simulink model "generic_truck"  (Simulink 8.7)
settings: Solver=ode45  StartTime=0.0  StopTime=inf  RelTol=1e-3
libraries: TruckMaker4SL x1, simulink x1
(part 1 of 2)
settings Model: Creator=fh  LastModifiedBy=IPG  ExtModeAutoUpdateStatusClock=off
settings DataIOCC: SignalLoggingSaveFormat=ModelDataLogs  SignalLoggingName=sigsOut
settings OptimizationCC: BooleanDataType=off  ExpressionDepthLimit=2147483647  InitFltsAndDblsToZero=on
settings DebuggingCC: SaveWithParameterizedLinksMsg=none  SignalResolutionControl=TryResolveAllWithWarning  MultiTaskDSMMsg=warning  MultiTaskCondExecSysMsg=none  FcnCallInpInsideContextMsg=UseLocalSettings  StateNameClashWarn=warning
settings HardwareCC: TargetUnknown=on
settings CodeAppCC: MaxIdLength=63
settings GRTTargetCC: TargetFcnLib=ansi_tfl_tmw.mat  CombineOutputUpdateFcns=off  GRTInterface=on

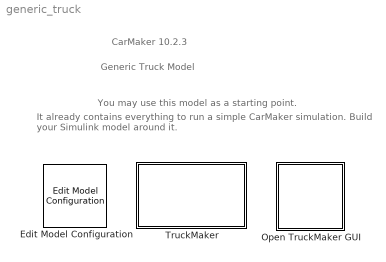
== system generic_truck ==
  note: Generic Truck Model
  note: CarMaker 10.2.3
  note: You may use this model as a starting point.
  note: It already contains everything to run a simple CarMaker simulation.
      | Build your Simulink model around it.
  Edit Model Configuration : TruckMaker4SL/Edit Model Configuration
  Open TruckMaker GUI : Subsystem  LoadFcn=if ~length(which('cmself')), cmenv; end
      settings: OpenFcn=cmblockmagic('gui_fix_display'); TM_Simulink
      mask Display: image(imread('TruckMakerGUI.png'));
  TruckMaker : Subsystem  TreatAsAtomicUnit=on
      mask Display: image(imread('TruckMakerSys.png'));

== system generic_truck/Open TruckMaker GUI ==
  S-Function : S-Function  FunctionName=cm_gui  SFunctionDeploymentMode=off  EnableBusSupport=off

== system generic_truck/TruckMaker ==
  CM_FIRST : Subsystem
  CM_LAST : Subsystem
  DrivMan : Subsystem
  Ground : Ground
  IPG Vehicle : Subsystem  TreatAsAtomicUnit=on
  Terminator : Terminator
  VehicleControl : Subsystem
  wires:
  VehicleControl/2(Vhcl.Model.Source) -> IPG Vehicle/2(Vhcl.Model.Source)
  VehicleControl/7(VhclCtrl.PT) -> IPG Vehicle/7(VhclCtrl.PT)
  VehicleControl/6(VhclCtrl.Brake) -> IPG Vehicle/6(VhclCtrl.Brake)
  VehicleControl/5(Vhcl.Misc) -> IPG Vehicle/5(Vhcl.Misc)
  VehicleControl/4(Vhcl.Wheel.In) -> IPG Vehicle/4(Vhcl.Wheel.In)
  VehicleControl/3(VhclCtrl.Steering) -> IPG Vehicle/3(VhclCtrl.Steering)
  VehicleControl/1(Sync_Out) -> IPG Vehicle/1(Sync_In)
  IPG Vehicle/1(Sync_Out) -> CM_LAST/1(Sync_In)
  Ground/1 -> CM_FIRST/1(Sync_In)
  CM_LAST/1(Sync_Out) -> Terminator/1
  CM_FIRST/1(Sync_Out) -> DrivMan/1(Sync_In)
  CM_FIRST/2(Env.Misc) -> DrivMan/2(Env.Misc)
  DrivMan/1(Sync_Out) -> VehicleControl/1(Sync_In)
  DrivMan/2(DrivMan.Out) -> VehicleControl/2(DrivMan.In)

== system generic_truck/TruckMaker/CM_FIRST ==
  Sync_In : Inport
  BusCreator1 : BusCreator  Inputs=8
  BusCreator2 : BusCreator  Inputs=6
  Demux1 : Demux  Outputs=14
  Environment : S-Function  FunctionName=TM_Sfun  Parameters='Environment'  SFunctionDeploymentMode=off  EnableBusSupport=off
  IoIn : S-Function  FunctionName=TM_Sfun  Parameters='IoIn'  SFunctionDeploymentMode=off  EnableBusSupport=off
  Terminator : Terminator
  Sync_Out : Outport
  Env.Misc : Outport  Port=2
  wires:
  BusCreator2/1 -> Terminator/1  "IF Environment (in)"
  BusCreator1/1 -> Env.Misc/1
  Demux1/14 -> BusCreator2/6  "Env sRoad"
  Demux1/13 -> BusCreator2/5  "Env PoI_GCS Elev"
  Demux1/12 -> BusCreator2/4  "Env PoI_GCS Lat"
  Demux1/11 -> BusCreator2/3  "Env PoI_GCS Long"
  Demux1/10 -> BusCreator2/2  "Env Time"
  Demux1/9 -> BusCreator2/1  "Env yDay"
  Demux1/8 -> BusCreator1/8  "Env WindVel_tot z"
  Demux1/7 -> BusCreator1/7  "Env WindVel_tot y"
  Demux1/6 -> BusCreator1/6  "Env WindVel_tot x"
  Demux1/5 -> BusCreator1/5  "Env SolarRadiation"
  Demux1/4 -> BusCreator1/4  "Env AirHumidity"
  Demux1/3 -> BusCreator1/3  "Env AirPressure"
  Demux1/2 -> BusCreator1/2  "Env AirDensity"
  Demux1/1 -> BusCreator1/1  "Env Temperature"
  Environment/2 -> Demux1/1
  Environment/1 -> Sync_Out/1
  IoIn/1 -> Environment/1
  Sync_In/1 -> IoIn/1

== system generic_truck/TruckMaker/CM_LAST ==
  Sync_In : Inport
  CM_User : S-Function  FunctionName=TM_Sfun  Parameters='CM_User'  SFunctionDeploymentMode=off  EnableBusSupport=off
  IoOut : S-Function  FunctionName=TM_Sfun  Parameters='IoOut'  SFunctionDeploymentMode=off  EnableBusSupport=off
  Sync_Out : Outport
  wires:
  IoOut/1 -> Sync_Out/1
  CM_User/1 -> IoOut/1
  Sync_In/1 -> CM_User/1

== system generic_truck/TruckMaker/DrivMan ==
  note: There's rarely a reason to override DrivMan signals.
      | Use the VehicleControl interface for this purpose.
  Sync_In : Inport
  Env.Misc : Inport  Port=2
  BusCreator : BusCreator  Inputs=17
  Demux : Demux  Outputs=17
  DrivMan : S-Function  FunctionName=TM_Sfun  Parameters='DrivMan'  SFunctionDeploymentMode=off  EnableBusSupport=off
  Sync_Out : Outport
  DrivMan.Out : Outport  Port=2
  wires:
  Demux/17 -> BusCreator/17  "DrivMan Steering Trq"
  Demux/16 -> BusCreator/16  "DrivMan Steering AngAcc"
  Demux/15 -> BusCreator/15  "DrivMan Steering AngVel"
  Demux/14 -> BusCreator/14  "DrivMan Steering Ang"
  Demux/13 -> BusCreator/13  "DrivMan Gas"
  Demux/12 -> BusCreator/12  "DrivMan Clutch"
  Demux/11 -> BusCreator/11  "DrivMan BrakePark"
  Demux/10 -> BusCreator/10  "DrivMan Brake"
  Demux/9 -> BusCreator/9  "DrivMan GearNo"
  Demux/8 -> BusCreator/8  "DrivMan SelectorCtrl"
  Demux/7 -> BusCreator/7  "DrivMan UserSignal4"
  Demux/6 -> BusCreator/6  "DrivMan UserSignal3"
  Demux/5 -> BusCreator/5  "DrivMan UserSignal2"
  Demux/4 -> BusCreator/4  "DrivMan UserSignal1"
  Demux/3 -> BusCreator/3  "DrivMan UserSignal0"
  Demux/2 -> BusCreator/2  "DrivMan Key"
  Demux/1 -> BusCreator/1  "DrivMan SST"
  Env.Misc/1 -> DrivMan/2
  Sync_In/1 -> DrivMan/1
  DrivMan/1 -> Sync_Out/1
  BusCreator/1 -> DrivMan.Out/1
  DrivMan/2 -> Demux/1

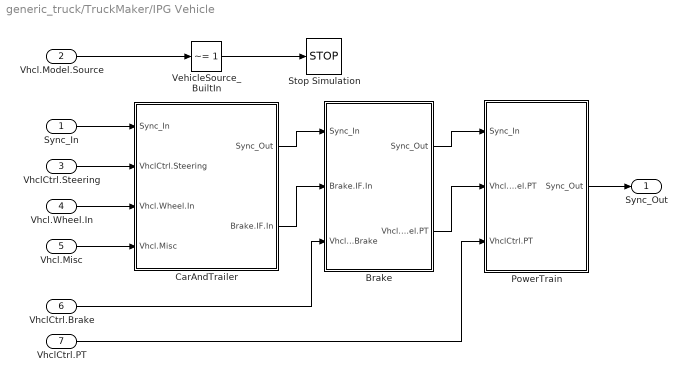
== system generic_truck/TruckMaker/IPG Vehicle ==
  Sync_In : Inport
  Vhcl.Model.Source : Inport  Port=2
  VhclCtrl.Steering : Inport  Port=3
  Vhcl.Wheel.In : Inport  Port=4
  Vhcl.Misc : Inport  Port=5
  VhclCtrl.Brake : Inport  Port=6
  VhclCtrl.PT : Inport  Port=7
  Brake : Subsystem
  CarAndTrailer : Subsystem
  PowerTrain : Subsystem
  Stop Simulation : Stop
  VehicleSource_BuiltIn : simulink/Logic and Bit Operations/Compare To Constant  relop=~=  const=1  OutDataTypeStr=boolean  ZeroCross=off
  Sync_Out : Outport
  wires:
  VhclCtrl.PT/1 -> PowerTrain/3(VhclCtrl.PT)
  Brake/1(Sync_Out) -> PowerTrain/1(Sync_In)
  CarAndTrailer/1(Sync_Out) -> Brake/1(Sync_In)
  CarAndTrailer/2(Brake.IF.In) -> Brake/2(Brake.IF.In)
  VhclCtrl.Brake/1 -> Brake/3(VhclCtrl.Brake)
  PowerTrain/1(Sync_Out) -> Sync_Out/1
  Vhcl.Misc/1 -> CarAndTrailer/4(Vhcl.Misc)
  Vhcl.Wheel.In/1 -> CarAndTrailer/3(Vhcl.Wheel.In)
  VhclCtrl.Steering/1 -> CarAndTrailer/2(VhclCtrl.Steering)
  Sync_In/1 -> CarAndTrailer/1(Sync_In)
  Vhcl.Model.Source/1 -> VehicleSource_BuiltIn/1
  VehicleSource_BuiltIn/1 -> Stop Simulation/1
  Brake/2(Vhcl.Wheel.PT) -> PowerTrain/2(Vhcl.Wheel.PT)

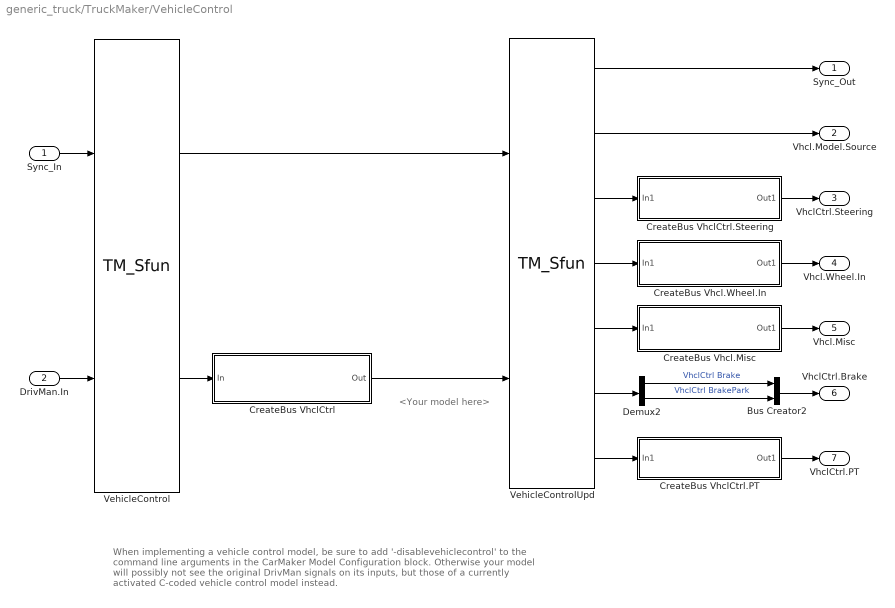
== system generic_truck/TruckMaker/VehicleControl ==
  note: <Your model here>
  note: When implementing a vehicle control model,
      | be sure to add '-disablevehiclecontrol' to the command line arguments
      | in the CarMaker Model Configuration block.
      | Otherwise your model will possibly not see the original DrivMan signals
      | on its inputs, but those of a currently activated C-coded vehicle control model instead.
  Sync_In : Inport
  DrivMan.In : Inport  Port=2
  Bus Creator2 : BusCreator  Inputs=2
  CreateBus Vhcl.Misc : Subsystem
  CreateBus Vhcl.Wheel.In : Subsystem
  CreateBus VhclCtrl : Subsystem
  CreateBus VhclCtrl.PT : Subsystem
  CreateBus VhclCtrl.Steering : Subsystem
  Demux2 : Demux  Outputs=2
  VehicleControl : S-Function  FunctionName=TM_Sfun  Parameters='VehicleControl'  SFunctionDeploymentMode=off  EnableBusSupport=off
  VehicleControlUpd : S-Function  FunctionName=TM_Sfun  Parameters='VehicleControlUpd'  SFunctionDeploymentMode=off  EnableBusSupport=off
  Sync_Out : Outport
  Vhcl.Model.Source : Outport  Port=2
  VhclCtrl.Steering : Outport  Port=3
  Vhcl.Wheel.In : Outport  Port=4
  Vhcl.Misc : Outport  Port=5
  VhclCtrl.Brake : Outport  Port=6
  VhclCtrl.PT : Outport  Port=7
  wires:
  VehicleControlUpd/2 -> Vhcl.Model.Source/1
  VehicleControlUpd/4 -> CreateBus Vhcl.Wheel.In/1(In1)
  VehicleControlUpd/5 -> CreateBus Vhcl.Misc/1(In1)
  VehicleControlUpd/6 -> Demux2/1
  VehicleControlUpd/7 -> CreateBus VhclCtrl.PT/1(In1)
  VehicleControlUpd/3 -> CreateBus VhclCtrl.Steering/1(In1)
  CreateBus Vhcl.Misc/1(Out1) -> Vhcl.Misc/1
  CreateBus Vhcl.Wheel.In/1(Out1) -> Vhcl.Wheel.In/1
  DrivMan.In/1 -> VehicleControl/2
  CreateBus VhclCtrl/1(Out) -> VehicleControlUpd/2
  VehicleControl/1 -> VehicleControlUpd/1
  VehicleControl/2 -> CreateBus VhclCtrl/1(In)
  Sync_In/1 -> VehicleControl/1
  CreateBus VhclCtrl.PT/1(Out1) -> VhclCtrl.PT/1
  Bus Creator2/1 -> VhclCtrl.Brake/1
  CreateBus VhclCtrl.Steering/1(Out1) -> VhclCtrl.Steering/1
  VehicleControlUpd/1 -> Sync_Out/1
  Demux2/2 -> Bus Creator2/2  "VhclCtrl BrakePark"
  Demux2/1 -> Bus Creator2/1  "VhclCtrl Brake"

== system generic_truck/TruckMaker/IPG Vehicle/Brake ==
  note: <Your model here>
  note: When replacing the entire braking system,
      | be sure to disable the IPG brake model by using the brake
      | model 'Model Manager off' in the vehicle GUI.
  Sync_In : Inport
  Brake.IF.In : Inport  Port=2
  VhclCtrl.Brake : Inport  Port=3
  Brake : S-Function  FunctionName=TM_Sfun  Parameters='Brake'  SFunctionDeploymentMode=off  EnableBusSupport=off
  BrakeUpd : S-Function  FunctionName=TM_Sfun  Parameters='BrakeUpd'  SFunctionDeploymentMode=off  EnableBusSupport=off
  BusCreator : BusCreator  Inputs=32
  CreateBus Vhcl.Wheel.PT : Subsystem
  Demux : Demux  Outputs=32
  Sync_Out : Outport
  Vhcl.Wheel.PT : Outport  Port=2
  wires:
  Demux/32 -> BusCreator/32  "Brake IF Trq_DriveSrc_trg d7"
  Demux/31 -> BusCreator/31  "Brake IF Trq_DriveSrc_trg d6"
  Demux/30 -> BusCreator/30  "Brake IF Trq_DriveSrc_trg d5"
  Demux/29 -> BusCreator/29  "Brake IF Trq_DriveSrc_trg d4"
  Demux/28 -> BusCreator/28  "Brake IF Trq_DriveSrc_trg d3"
  Demux/27 -> BusCreator/27  "Brake IF Trq_DriveSrc_trg d2"
  Demux/26 -> BusCreator/26  "Brake IF Trq_DriveSrc_trg d1"
  Demux/25 -> BusCreator/25  "Brake IF Trq_DriveSrc_trg d0"
  Demux/24 -> BusCreator/24  "Brake IF Trq_Reg_trg FR2"
  Demux/23 -> BusCreator/23  "Brake IF Trq_Reg_trg FL2"
  Demux/22 -> BusCreator/22  "Brake IF Trq_Reg_trg RR2"
  Demux/21 -> BusCreator/21  "Brake IF Trq_Reg_trg RL2"
  Demux/20 -> BusCreator/20  "Brake IF Trq_Reg_trg RR"
  Demux/19 -> BusCreator/19  "Brake IF Trq_Reg_trg RL"
  Demux/18 -> BusCreator/18  "Brake IF Trq_Reg_trg FR"
  Demux/17 -> BusCreator/17  "Brake IF Trq_Reg_trg FL"
  Demux/16 -> BusCreator/16  "Brake IF Trq_PB FR2"
  Demux/15 -> BusCreator/15  "Brake IF Trq_PB FL2"
  Demux/14 -> BusCreator/14  "Brake IF Trq_PB RR2"
  Demux/13 -> BusCreator/13  "Brake IF Trq_PB RL2"
  Demux/12 -> BusCreator/12  "Brake IF Trq_PB RR"
  Demux/11 -> BusCreator/11  "Brake IF Trq_PB RL"
  Demux/10 -> BusCreator/10  "Brake IF Trq_PB FR"
  Demux/9 -> BusCreator/9  "Brake IF Trq_PB FL"
  Demux/8 -> BusCreator/8  "Brake IF Trq_WB FR2"
  Demux/7 -> BusCreator/7  "Brake IF Trq_WB FL2"
  Demux/6 -> BusCreator/6  "Brake IF Trq_WB RR2"
  Demux/5 -> BusCreator/5  "Brake IF Trq_WB RL2"
  Demux/4 -> BusCreator/4  "Brake IF Trq_WB RR"
  Demux/3 -> BusCreator/3  "Brake IF Trq_WB RL"
  Demux/2 -> BusCreator/2  "Brake IF Trq_WB FR"
  Demux/1 -> BusCreator/1  "Brake IF Trq_WB FL"
  BusCreator/1 -> BrakeUpd/2
  Brake/2 -> Demux/1
  BrakeUpd/1 -> Sync_Out/1
  Brake/1 -> BrakeUpd/1  "Sync"
  Brake.IF.In/1 -> Brake/2
  VhclCtrl.Brake/1 -> Brake/3
  Sync_In/1 -> Brake/1
  BrakeUpd/2 -> CreateBus Vhcl.Wheel.PT/1(In)
  CreateBus Vhcl.Wheel.PT/1(Out) -> Vhcl.Wheel.PT/1

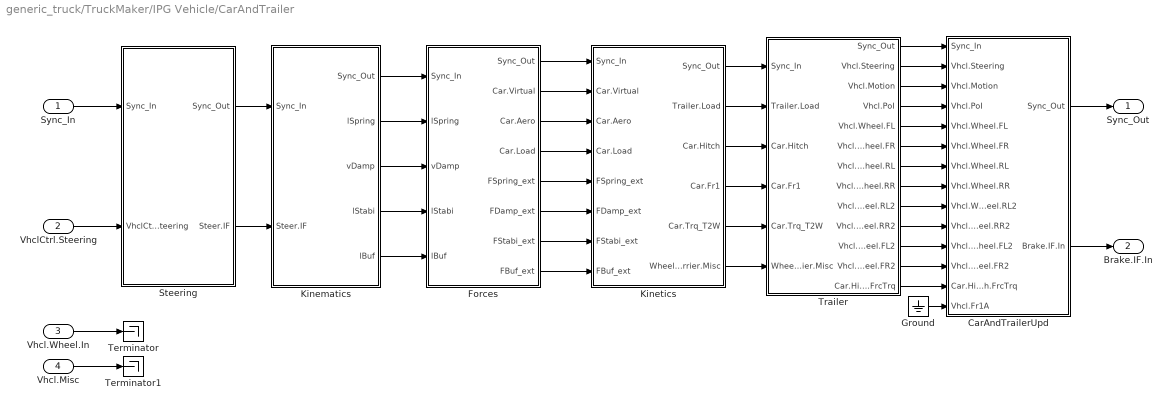
== system generic_truck/TruckMaker/IPG Vehicle/CarAndTrailer ==
  Sync_In : Inport
  VhclCtrl.Steering : Inport  Port=2
  Vhcl.Wheel.In : Inport  Port=3
  Vhcl.Misc : Inport  Port=4
  CarAndTrailerUpd : Subsystem
  Forces : Subsystem
  Ground : Ground
  Kinematics : Subsystem
  Kinetics : Subsystem
  Steering : Subsystem
  Terminator : Terminator
  Terminator1 : Terminator
  Trailer : Subsystem
  Sync_Out : Outport
  Brake.IF.In : Outport  Port=2
  wires:
  Ground/1 -> CarAndTrailerUpd/14(Vhcl.Fr1A)
  Trailer/13(Car.Hitch.FrcTrq) -> CarAndTrailerUpd/13(Car.Hitch.FrcTrq)
  Trailer/12(Vhcl.Wheel.FR2) -> CarAndTrailerUpd/12(Vhcl.Wheel.FR2)
  Trailer/11(Vhcl.Wheel.FL2) -> CarAndTrailerUpd/11(Vhcl.Wheel.FL2)
  Trailer/10(Vhcl.Wheel.RR2) -> CarAndTrailerUpd/10(Vhcl.Wheel.RR2)
  Trailer/9(Vhcl.Wheel.RL2) -> CarAndTrailerUpd/9(Vhcl.Wheel.RL2)
  Trailer/8(Vhcl.Wheel.RR) -> CarAndTrailerUpd/8(Vhcl.Wheel.RR)
  Trailer/7(Vhcl.Wheel.RL) -> CarAndTrailerUpd/7(Vhcl.Wheel.RL)
  Trailer/6(Vhcl.Wheel.FR) -> CarAndTrailerUpd/6(Vhcl.Wheel.FR)
  Trailer/5(Vhcl.Wheel.FL) -> CarAndTrailerUpd/5(Vhcl.Wheel.FL)
  Trailer/4(Vhcl.PoI) -> CarAndTrailerUpd/4(Vhcl.PoI)
  Trailer/3(Vhcl.Motion) -> CarAndTrailerUpd/3(Vhcl.Motion)
  Trailer/2(Vhcl.Steering) -> CarAndTrailerUpd/2(Vhcl.Steering)
  Trailer/1(Sync_Out) -> CarAndTrailerUpd/1(Sync_In)
  CarAndTrailerUpd/2(Brake.IF.In) -> Brake.IF.In/1
  CarAndTrailerUpd/1(Sync_Out) -> Sync_Out/1
  Vhcl.Misc/1 -> Terminator1/1
  Vhcl.Wheel.In/1 -> Terminator/1
  Kinetics/6(WheelCarrier.Misc) -> Trailer/6(WheelCarrier.Misc)
  Kinetics/5(Car.Trq_T2W) -> Trailer/5(Car.Trq_T2W)
  Steering/2(Steer.IF) -> Kinematics/2(Steer.IF)
  Kinetics/4(Car.Fr1) -> Trailer/4(Car.Fr1)
  Kinetics/3(Car.Hitch) -> Trailer/3(Car.Hitch)
  Kinetics/2(Trailer.Load) -> Trailer/2(Trailer.Load)
  VhclCtrl.Steering/1 -> Steering/2(VhclCtrl.Steering)
  Sync_In/1 -> Steering/1(Sync_In)
  Steering/1(Sync_Out) -> Kinematics/1(Sync_In)
  Kinetics/1(Sync_Out) -> Trailer/1(Sync_In)
  Kinematics/5(lBuf) -> Forces/5(lBuf)
  Forces/8(FBuf_ext) -> Kinetics/8(FBuf_ext)
  Forces/4(Car.Load) -> Kinetics/4(Car.Load)
  Forces/7(FStabi_ext) -> Kinetics/7(FStabi_ext)
  Forces/6(FDamp_ext) -> Kinetics/6(FDamp_ext)
  Forces/5(FSpring_ext) -> Kinetics/5(FSpring_ext)
  Forces/2(Car.Virtual) -> Kinetics/2(Car.Virtual)
  Kinematics/2(lSpring) -> Forces/2(lSpring)
  Kinematics/3(vDamp) -> Forces/3(vDamp)
  Forces/3(Car.Aero) -> Kinetics/3(Car.Aero)
  Forces/1(Sync_Out) -> Kinetics/1(Sync_In)
  Kinematics/1(Sync_Out) -> Forces/1(Sync_In)
  Kinematics/4(lStabi) -> Forces/4(lStabi)

== system generic_truck/TruckMaker/IPG Vehicle/PowerTrain ==
  note: When replacing the entire powertrain,
      | be sure to disable the IPG powertrain model by using the powertrain
      | model 'Model Manager off' in the vehicle GUI.
  note: <Your model here>
  Sync_In : Inport
  Vhcl.Wheel.PT : Inport  Port=2
  VhclCtrl.PT : Inport  Port=3
  BusCreator : BusCreator  Inputs=70
  Demux : Demux  Outputs=70
  PowerTrain : S-Function  FunctionName=TM_Sfun  Parameters='PowerTrain'  SFunctionDeploymentMode=off  EnableBusSupport=off
  PowerTrainUpd : S-Function  FunctionName=TM_Sfun  Parameters='PowerTrainUpd'  SFunctionDeploymentMode=off  EnableBusSupport=off
  Sync_Out : Outport
  wires:
  Demux/70 -> BusCreator/70  "PT IF WFR2 Trq_BrakeReg_max"
  Demux/69 -> BusCreator/69  "PT IF WFR2 Trq_BrakeReg"
  Demux/68 -> BusCreator/68  "PT IF WFR2 Trq_Supp2WC"
  Demux/67 -> BusCreator/67  "PT IF WFR2 Trq_Drive"
  Demux/66 -> BusCreator/66  "PT IF WFR2 Trq_B2W"
  Demux/65 -> BusCreator/65  "PT IF WFR2 rotv"
  Demux/64 -> BusCreator/64  "PT IF WFR2 rot"
  Demux/63 -> BusCreator/63  "PT IF WFL2 Trq_BrakeReg_max"
  Demux/62 -> BusCreator/62  "PT IF WFL2 Trq_BrakeReg"
  Demux/61 -> BusCreator/61  "PT IF WFL2 Trq_Supp2WC"
  Demux/60 -> BusCreator/60  "PT IF WFL2 Trq_Drive"
  Demux/59 -> BusCreator/59  "PT IF WFL2 Trq_B2W"
  Demux/58 -> BusCreator/58  "PT IF WFL2 rotv"
  Demux/57 -> BusCreator/57  "PT IF WFL2 rot"
  Demux/56 -> BusCreator/56  "PT IF WRR2 Trq_BrakeReg_max"
  Demux/55 -> BusCreator/55  "PT IF WRR2 Trq_BrakeReg"
  Demux/54 -> BusCreator/54  "PT IF WRR2 Trq_Supp2WC"
  Demux/53 -> BusCreator/53  "PT IF WRR2 Trq_Drive"
  Demux/52 -> BusCreator/52  "PT IF WRR2 Trq_B2W"
  Demux/51 -> BusCreator/51  "PT IF WRR2 rotv"
  Demux/50 -> BusCreator/50  "PT IF WRR2 rot"
  Demux/49 -> BusCreator/49  "PT IF WRL2 Trq_BrakeReg_max"
  Demux/48 -> BusCreator/48  "PT IF WRL2 Trq_BrakeReg"
  Demux/47 -> BusCreator/47  "PT IF WRL2 Trq_Supp2WC"
  Demux/46 -> BusCreator/46  "PT IF WRL2 Trq_Drive"
  Demux/45 -> BusCreator/45  "PT IF WRL2 Trq_B2W"
  Demux/44 -> BusCreator/44  "PT IF WRL2 rotv"
  Demux/43 -> BusCreator/43  "PT IF WRL2 rot"
  Demux/42 -> BusCreator/42  "PT IF WRR Trq_BrakeReg_max"
  Demux/41 -> BusCreator/41  "PT IF WRR Trq_BrakeReg"
  Demux/40 -> BusCreator/40  "PT IF WRR Trq_Supp2WC"
  Demux/39 -> BusCreator/39  "PT IF WRR Trq_Drive"
  Demux/38 -> BusCreator/38  "PT IF WRR Trq_B2W"
  Demux/37 -> BusCreator/37  "PT IF WRR rotv"
  Demux/36 -> BusCreator/36  "PT IF WRR rot"
  Demux/35 -> BusCreator/35  "PT IF WRL Trq_BrakeReg_max"
  Demux/34 -> BusCreator/34  "PT IF WRL Trq_BrakeReg"
  Demux/33 -> BusCreator/33  "PT IF WRL Trq_Supp2WC"
  Demux/32 -> BusCreator/32  "PT IF WRL Trq_Drive"
  Demux/31 -> BusCreator/31  "PT IF WRL Trq_B2W"
  Demux/30 -> BusCreator/30  "PT IF WRL rotv"
  Demux/29 -> BusCreator/29  "PT IF WRL rot"
  Demux/28 -> BusCreator/28  "PT IF WFR Trq_BrakeReg_max"
  Demux/27 -> BusCreator/27  "PT IF WFR Trq_BrakeReg"
  Demux/26 -> BusCreator/26  "PT IF WFR Trq_Supp2WC"
  Demux/25 -> BusCreator/25  "PT IF WFR Trq_Drive"
  Demux/24 -> BusCreator/24  "PT IF WFR Trq_B2W"
  Demux/23 -> BusCreator/23  "PT IF WFR rotv"
  Demux/22 -> BusCreator/22  "PT IF WFR rot"
  Demux/21 -> BusCreator/21  "PT IF WFL Trq_BrakeReg_max"
  Demux/20 -> BusCreator/20  "PT IF WFL Trq_BrakeReg"
  Demux/19 -> BusCreator/19  "PT IF WFL Trq_Supp2WC"
  Demux/18 -> BusCreator/18  "PT IF WFL Trq_Drive"
  Demux/17 -> BusCreator/17  "PT IF WFL Trq_B2W"
  Demux/16 -> BusCreator/16  "PT IF WFL rotv"
  Demux/15 -> BusCreator/15  "PT IF WFL rot"
  Demux/14 -> BusCreator/14  "PT IF DL_iDiff_mean"
  Demux/13 -> BusCreator/13  "PT IF Trq_Supp2BdyEng y"
  Demux/12 -> BusCreator/12  "PT IF Trq_Supp2BdyEng x"
  Demux/11 -> BusCreator/11  "PT IF Trq_Supp2Bdy1B z"
  Demux/10 -> BusCreator/10  "PT IF Trq_Supp2Bdy1B y"
  Demux/9 -> BusCreator/9  "PT IF Trq_Supp2Bdy1B x"
  Demux/8 -> BusCreator/8  "PT IF Trq_Supp2Bdy1 z"
  Demux/7 -> BusCreator/7  "PT IF Trq_Supp2Bdy1 y"
  Demux/6 -> BusCreator/6  "PT IF Trq_Supp2Bdy1 x"
  Demux/5 -> BusCreator/5  "PT IF Engine_rotv"
  Demux/4 -> BusCreator/4  "PT IF GearNo"
  Demux/3 -> BusCreator/3  "PT IF OperationError"
  Demux/2 -> BusCreator/2  "PT IF OperationState"
  Demux/1 -> BusCreator/1  "PT IF Ignition"
  BusCreator/1 -> PowerTrainUpd/2
  PowerTrain/2 -> Demux/1
  Sync_In/1 -> PowerTrain/1
  PowerTrainUpd/1 -> Sync_Out/1
  PowerTrain/1 -> PowerTrainUpd/1  "Sync"
  VhclCtrl.PT/1 -> PowerTrain/3
  Vhcl.Wheel.PT/1 -> PowerTrain/2

== system generic_truck/TruckMaker/VehicleControl/CreateBus Vhcl.Misc ==
  In1 : Inport
  Bus Creator5 : BusCreator  Inputs=11
  Demux5 : Demux  Outputs=11
  Out1 : Outport
  wires:
  Demux5/11 -> Bus Creator5/11  "Vhcl Wind_vel_0 z"
  Demux5/10 -> Bus Creator5/10  "Vhcl Wind_vel_0 y"
  Demux5/9 -> Bus Creator5/9  "Vhcl Wind_vel_0 x"
  Demux5/8 -> Bus Creator5/8  "Vhcl DL2BdyEng y"
  Demux5/7 -> Bus Creator5/7  "Vhcl DL2BdyEng x"
  Demux5/6 -> Bus Creator5/6  "Vhcl TrqDL2Bdy1B z"
  Demux5/5 -> Bus Creator5/5  "Vhcl TrqDL2Bdy1B y"
  Demux5/4 -> Bus Creator5/4  "Vhcl TrqDL2Bdy1B x"
  Demux5/3 -> Bus Creator5/3  "Vhcl Trq_DL2Bdy1 z"
  In1/1 -> Demux5/1
  Bus Creator5/1 -> Out1/1
  Demux5/2 -> Bus Creator5/2  "Vhcl Trq_DL2Bdy1 y"
  Demux5/1 -> Bus Creator5/1  "Vhcl Trq_DL2Bdy1 x"

== system generic_truck/TruckMaker/VehicleControl/CreateBus Vhcl.Wheel.In ==
  In1 : Inport
  Bus Creator1 : BusCreator  Inputs=24
  Demux1 : Demux  Outputs=24
  Out1 : Outport
  wires:
  Demux1/12 -> Bus Creator1/12  "Vhcl Wheel RR rotv"
  Demux1/11 -> Bus Creator1/11  "Vhcl Wheel RR Trq_DL2WC"
  Demux1/10 -> Bus Creator1/10  "Vhcl Wheel RR Trq_B2WC"
  Demux1/9 -> Bus Creator1/9  "Vhcl Wheel RL rotv"
  Demux1/8 -> Bus Creator1/8  "Vhcl Wheel RL Trq_DL2WC"
  Demux1/7 -> Bus Creator1/7  "Vhcl Wheel RL Trq_B2WC"
  Demux1/6 -> Bus Creator1/6  "Vhcl Wheel FR rotv"
  Demux1/5 -> Bus Creator1/5  "Vhcl Wheel FR Trq_DL2WC"
  Demux1/4 -> Bus Creator1/4  "Vhcl Wheel FR Trq_B2WC"
  Demux1/3 -> Bus Creator1/3  "Vhcl Wheel FL rotv"
  Demux1/2 -> Bus Creator1/2  "Vhcl Wheel FL Trq_DL2WC"
  Demux1/1 -> Bus Creator1/1  "Vhcl Wheel FL Trq_B2WC"
  Bus Creator1/1 -> Out1/1
  In1/1 -> Demux1/1
  Demux1/24 -> Bus Creator1/24  "Vhcl Wheel FR2 rotv"
  Demux1/23 -> Bus Creator1/23  "Vhcl Wheel FR2 Trq_DL2WC"
  Demux1/22 -> Bus Creator1/22  "Vhcl Wheel FR2 Trq_B2WC"
  Demux1/21 -> Bus Creator1/21  "Vhcl Wheel FL2 rotv"
  Demux1/20 -> Bus Creator1/20  "Vhcl Wheel FL2 Trq_DL2WC"
  Demux1/19 -> Bus Creator1/19  "Vhcl Wheel FL2 Trq_B2WC"
  Demux1/18 -> Bus Creator1/18  "Vhcl Wheel RR2 rotv"
  Demux1/17 -> Bus Creator1/17  "Vhcl Wheel RR2 Trq_DL2WC"
  Demux1/16 -> Bus Creator1/16  "Vhcl Wheel RR2 Trq_B2WC"
  Demux1/15 -> Bus Creator1/15  "Vhcl Wheel RL2 rotv"
  Demux1/14 -> Bus Creator1/14  "Vhcl Wheel RL2 Trq_DL2WC"
  Demux1/13 -> Bus Creator1/13  "Vhcl Wheel RL2 Trq_B2WC"

== system generic_truck/TruckMaker/VehicleControl/CreateBus VhclCtrl ==
  In : Inport
  BusCreator : BusCreator  Inputs=29
  Demux : Demux  Outputs=29
  Out : Outport
  wires:
  Demux/29 -> BusCreator/29  "VhclCtrl Lights Reverse"
  Demux/28 -> BusCreator/28  "VhclCtrl Lights Brake"
  Demux/27 -> BusCreator/27  "VhclCtrl Lights FogRear"
  Demux/26 -> BusCreator/26  "VhclCtrl Lights FogFrontR"
  Demux/25 -> BusCreator/25  "VhclCtrl Lights FogFrontL"
  Demux/24 -> BusCreator/24  "VhclCtrl Lights IndR"
  Demux/23 -> BusCreator/23  "VhclCtrl Lights IndL"
  Demux/22 -> BusCreator/22  "VhclCtrl Lights ParkR"
  Demux/21 -> BusCreator/21  "VhclCtrl Lights ParkL"
  Demux/20 -> BusCreator/20  "VhclCtrl Lights Daytime"
  Demux/19 -> BusCreator/19  "VhclCtrl Lights HighBeam"
  Demux/18 -> BusCreator/18  "VhclCtrl Lights LowBeam"
  Demux/17 -> BusCreator/17  "VhclCtrl Steering Trq"
  Demux/16 -> BusCreator/16  "VhclCtrl Steering AngAcc"
  Demux/15 -> BusCreator/15  "VhclCtrl Steering AngVel"
  Demux/14 -> BusCreator/14  "VhclCtrl Steering Ang"
  Demux/13 -> BusCreator/13  "VhclCtrl Gas"
  Demux/12 -> BusCreator/12  "VhclCtrl Clutch"
  Demux/11 -> BusCreator/11  "VhclCtrl BrakePark"
  Demux/10 -> BusCreator/10  "VhclCtrl Brake"
  Demux/9 -> BusCreator/9  "VhclCtrl SelectorCtrl"
  Demux/8 -> BusCreator/8  "VhclCtrl GearNo"
  Demux/7 -> BusCreator/7  "VhclCtrl UserSignal4"
  Demux/6 -> BusCreator/6  "VhclCtrl UserSignal3"
  Demux/5 -> BusCreator/5  "VhclCtrl UserSignal2"
  Demux/4 -> BusCreator/4  "VhclCtrl UserSignal1"
  Demux/3 -> BusCreator/3  "VhclCtrl UserSignal0"
  Demux/2 -> BusCreator/2  "VhclCtrl Key"
  Demux/1 -> BusCreator/1  "VhclCtrl SST"
  BusCreator/1 -> Out/1
  In/1 -> Demux/1

== system generic_truck/TruckMaker/VehicleControl/CreateBus VhclCtrl.PT ==
  In1 : Inport
  BusCreator1 : BusCreator  Inputs=12
  Demux1 : Demux  Outputs=12
  Out1 : Outport
  wires:
  BusCreator1/1 -> Out1/1
  In1/1 -> Demux1/1
  Demux1/1 -> BusCreator1/1  "VhclCtrl SST"
  Demux1/2 -> BusCreator1/2  "VhclCtrl Key"
  Demux1/3 -> BusCreator1/3  "VhclCtrl UserSignal0"
  Demux1/4 -> BusCreator1/4  "VhclCtrl UserSignal1"
  Demux1/5 -> BusCreator1/5  "VhclCtrl UserSignal2"
  Demux1/6 -> BusCreator1/6  "VhclCtrl UserSignal3"
  Demux1/7 -> BusCreator1/7  "VhclCtrl UserSignal4"
  Demux1/8 -> BusCreator1/8  "VhclCtrl GearNo"
  Demux1/9 -> BusCreator1/9  "VhclCtrl SelectorCtrl"
  Demux1/10 -> BusCreator1/10  "VhclCtrl Clutch"
  Demux1/11 -> BusCreator1/11  "VhclCtrl Gas"
  Demux1/12 -> BusCreator1/12  "VhclCtrl Brake"

== system generic_truck/TruckMaker/VehicleControl/CreateBus VhclCtrl.Steering ==
  In1 : Inport
  Bus Creator : BusCreator  Inputs=5
  Demux : Demux  Outputs=5
  Out1 : Outport
  wires:
  In1/1 -> Demux/1
  Bus Creator/1 -> Out1/1
  Demux/1 -> Bus Creator/1  "VhclCtrl Steering Ang"
  Demux/5 -> Bus Creator/5  "VhclCtrl Steering ByTrq"
  Demux/3 -> Bus Creator/3  "VhclCtrl Steering AngAcc"
  Demux/2 -> Bus Creator/2  "VhclCtrl Steering AngVel"
  Demux/4 -> Bus Creator/4  "VhclCtrl Steering Trq"

== system generic_truck/TruckMaker/IPG Vehicle/Brake/CreateBus Vhcl.Wheel.PT ==
  In : Inport
  BusCreator : BusCreator  Inputs=40
  Demux : Demux  Outputs=40
  Out : Outport
  wires:
  Demux/40 -> BusCreator/40  "Vhcl Trq_DriveSrc_trg d7"
  Demux/39 -> BusCreator/39  "Vhcl Trq_DriveSrc_trg d6"
  Demux/38 -> BusCreator/38  "Vhcl Trq_DriveSrc_trg d5"
  Demux/37 -> BusCreator/37  "Vhcl Trq_DriveSrc_trg d4"
  Demux/36 -> BusCreator/36  "Vhcl Trq_DriveSrc_trg d3"
  Demux/35 -> BusCreator/35  "Vhcl Trq_DriveSrc_trg d2"
  Demux/34 -> BusCreator/34  "Vhcl Trq_DriveSrc_trg d1"
  Demux/33 -> BusCreator/33  "Vhcl Trq_DriveSrc_trg d0"
  Demux/32 -> BusCreator/32  "Vhcl Wheel FR2 WhlBearing"
  Demux/31 -> BusCreator/31  "Vhcl Wheel FR2 Trq_T2W"
  Demux/30 -> BusCreator/30  "Vhcl Wheel FR2 Trq_BrakeReg_trg"
  Demux/29 -> BusCreator/29  "Vhcl Wheel FR2 Trq_Brake"
  Demux/28 -> BusCreator/28  "Vhcl Wheel FL2 WhlBearing"
  Demux/27 -> BusCreator/27  "Vhcl Wheel FL2 Trq_T2W"
  Demux/26 -> BusCreator/26  "Vhcl Wheel FL2 Trq_BrakeReg_trg"
  Demux/25 -> BusCreator/25  "Vhcl Wheel FL2 Trq_Brake"
  Demux/24 -> BusCreator/24  "Vhcl Wheel RR2 WhlBearing"
  Demux/23 -> BusCreator/23  "Vhcl Wheel RR2 Trq_T2W"
  Demux/22 -> BusCreator/22  "Vhcl Wheel RR2 Trq_BrakeReg_trg"
  Demux/21 -> BusCreator/21  "Vhcl Wheel RR2 Trq_Brake"
  Demux/20 -> BusCreator/20  "Vhcl Wheel RL2 WhlBearing"
  Demux/19 -> BusCreator/19  "Vhcl Wheel RL2 Trq_T2W"
  Demux/18 -> BusCreator/18  "Vhcl Wheel RL2 Trq_BrakeReg_trg"
  Demux/17 -> BusCreator/17  "Vhcl Wheel RL2 Trq_Brake"
  Demux/16 -> BusCreator/16  "Vhcl Wheel RR WhlBearing"
  Demux/15 -> BusCreator/15  "Vhcl Wheel RR Trq_T2W"
  Demux/14 -> BusCreator/14  "Vhcl Wheel RR Trq_BrakeReg_trg"
  Demux/13 -> BusCreator/13  "Vhcl Wheel RR Trq_Brake"
  Demux/12 -> BusCreator/12  "Vhcl Wheel RL WhlBearing"
  Demux/11 -> BusCreator/11  "Vhcl Wheel RL Trq_T2W"
  Demux/10 -> BusCreator/10  "Vhcl Wheel RL Trq_BrakeReg_trg"
  Demux/9 -> BusCreator/9  "Vhcl Wheel RL Trq_Brake"
  Demux/8 -> BusCreator/8  "Vhcl Wheel FR WhlBearing"
  Demux/7 -> BusCreator/7  "Vhcl Wheel FR Trq_T2W"
  Demux/6 -> BusCreator/6  "Vhcl Wheel FR Trq_BrakeReg_trg"
  Demux/5 -> BusCreator/5  "Vhcl Wheel FR Trq_Brake"
  Demux/4 -> BusCreator/4  "Vhcl Wheel FL WhlBearing"
  Demux/3 -> BusCreator/3  "Vhcl Wheel FL Trq_T2W"
  Demux/2 -> BusCreator/2  "Vhcl Wheel FL Trq_BrakeReg_trg"
  Demux/1 -> BusCreator/1  "Vhcl Wheel FL Trq_Brake"
  BusCreator/1 -> Out/1
  In/1 -> Demux/1

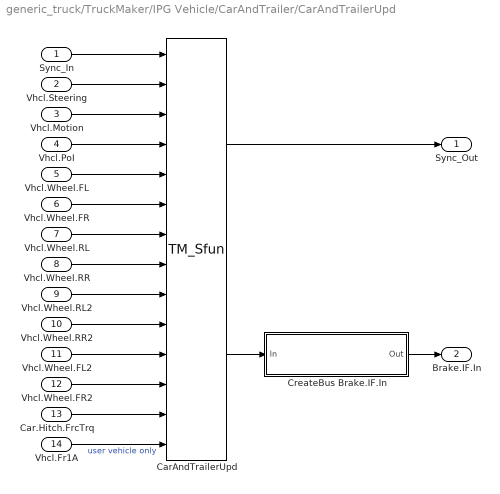
== system generic_truck/TruckMaker/IPG Vehicle/CarAndTrailer/CarAndTrailerUpd ==
  Sync_In : Inport
  Vhcl.Steering : Inport  Port=2
  Vhcl.Motion : Inport  Port=3
  Vhcl.PoI : Inport  Port=4
  Vhcl.Wheel.FL : Inport  Port=5
  Vhcl.Wheel.FR : Inport  Port=6
  Vhcl.Wheel.RL : Inport  Port=7
  Vhcl.Wheel.RR : Inport  Port=8
  Vhcl.Wheel.RL2 : Inport  Port=9
  Vhcl.Wheel.RR2 : Inport  Port=10
  Vhcl.Wheel.FL2 : Inport  Port=11
  Vhcl.Wheel.FR2 : Inport  Port=12
  Car.Hitch.FrcTrq : Inport  Port=13
  Vhcl.Fr1A : Inport  Port=14
  CarAndTrailerUpd : S-Function  FunctionName=TM_Sfun  Parameters='CarAndTrUpd'  SFunctionDeploymentMode=off  EnableBusSupport=off
  CreateBus Brake.IF.In : Subsystem
  Sync_Out : Outport
  Brake.IF.In : Outport  Port=2
  wires:
  Vhcl.Fr1A/1 -> CarAndTrailerUpd/14  "user vehicle only"
  Vhcl.Wheel.RL2/1 -> CarAndTrailerUpd/9
  Vhcl.Wheel.RR2/1 -> CarAndTrailerUpd/10
  Vhcl.Wheel.FL2/1 -> CarAndTrailerUpd/11
  Vhcl.Wheel.FR2/1 -> CarAndTrailerUpd/12
  Car.Hitch.FrcTrq/1 -> CarAndTrailerUpd/13
  Vhcl.Wheel.RR/1 -> CarAndTrailerUpd/8
  Vhcl.Wheel.RL/1 -> CarAndTrailerUpd/7
  Vhcl.Wheel.FR/1 -> CarAndTrailerUpd/6
  Vhcl.Wheel.FL/1 -> CarAndTrailerUpd/5
  Vhcl.Steering/1 -> CarAndTrailerUpd/2
  Vhcl.Motion/1 -> CarAndTrailerUpd/3
  Vhcl.PoI/1 -> CarAndTrailerUpd/4
  CarAndTrailerUpd/2 -> CreateBus Brake.IF.In/1(In)
  CreateBus Brake.IF.In/1(Out) -> Brake.IF.In/1
  CarAndTrailerUpd/1 -> Sync_Out/1
  Sync_In/1 -> CarAndTrailerUpd/1

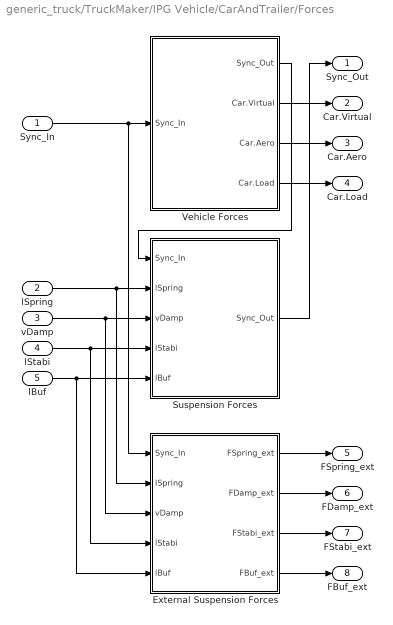
== system generic_truck/TruckMaker/IPG Vehicle/CarAndTrailer/Forces ==
  Sync_In : Inport
  lSpring : Inport  Port=2
  vDamp : Inport  Port=3
  lStabi : Inport  Port=4
  lBuf : Inport  Port=5
  External Suspension Forces : Subsystem
  Suspension Forces : Subsystem
  Vehicle Forces : Subsystem
  Sync_Out : Outport
  Car.Virtual : Outport  Port=2
  Car.Aero : Outport  Port=3
  Car.Load : Outport  Port=4
  FSpring_ext : Outport  Port=5
  FDamp_ext : Outport  Port=6
  FStabi_ext : Outport  Port=7
  FBuf_ext : Outport  Port=8
  wires:
  Sync_In/1 -> External Suspension Forces/1(Sync_In), Vehicle Forces/1(Sync_In)
  Vehicle Forces/2(Car.Virtual) -> Car.Virtual/1
  Vehicle Forces/3(Car.Aero) -> Car.Aero/1
  Vehicle Forces/4(Car.Load) -> Car.Load/1
  lSpring/1 -> Suspension Forces/2(lSpring), External Suspension Forces/2(lSpring)
  External Suspension Forces/2(FDamp_ext) -> FDamp_ext/1
  vDamp/1 -> Suspension Forces/3(vDamp), External Suspension Forces/3(vDamp)
  lStabi/1 -> Suspension Forces/4(lStabi), External Suspension Forces/4(lStabi)
  External Suspension Forces/3(FStabi_ext) -> FStabi_ext/1
  External Suspension Forces/1(FSpring_ext) -> FSpring_ext/1
  lBuf/1 -> Suspension Forces/5(lBuf), External Suspension Forces/5(lBuf)
  External Suspension Forces/4(FBuf_ext) -> FBuf_ext/1
  Vehicle Forces/1(Sync_Out) -> Suspension Forces/1(Sync_In)
  Suspension Forces/1(Sync_Out) -> Sync_Out/1

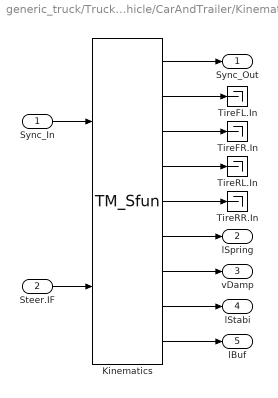
== system generic_truck/TruckMaker/IPG Vehicle/CarAndTrailer/Kinematics ==
  Sync_In : Inport
  Steer.IF : Inport  Port=2
  Kinematics : S-Function  FunctionName=TM_Sfun  Parameters='Kinematics'  SFunctionDeploymentMode=off  EnableBusSupport=off
  TireFL.In : Terminator
  TireFR.In : Terminator
  TireRL.In : Terminator
  TireRR.In : Terminator
  Sync_Out : Outport
  lSpring : Outport  Port=2
  vDamp : Outport  Port=3
  lStabi : Outport  Port=4
  lBuf : Outport  Port=5
  wires:
  Kinematics/8 -> lStabi/1
  Kinematics/2 -> TireFL.In/1
  Kinematics/3 -> TireFR.In/1
  Kinematics/4 -> TireRL.In/1
  Kinematics/5 -> TireRR.In/1
  Kinematics/6 -> lSpring/1
  Kinematics/7 -> vDamp/1
  Sync_In/1 -> Kinematics/1
  Kinematics/1 -> Sync_Out/1
  Steer.IF/1 -> Kinematics/2
  Kinematics/9 -> lBuf/1

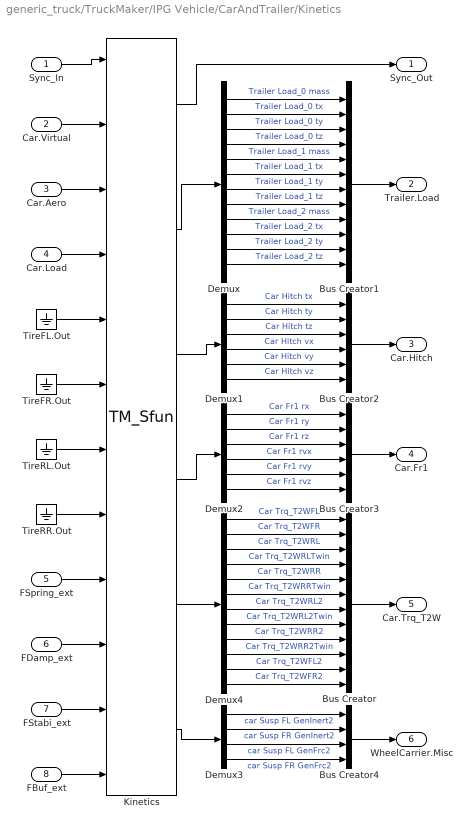
== system generic_truck/TruckMaker/IPG Vehicle/CarAndTrailer/Kinetics ==
  Sync_In : Inport
  Car.Virtual : Inport  Port=2
  Car.Aero : Inport  Port=3
  Car.Load : Inport  Port=4
  FSpring_ext : Inport  Port=5
  FDamp_ext : Inport  Port=6
  FStabi_ext : Inport  Port=7
  FBuf_ext : Inport  Port=8
  Bus Creator : BusCreator  Inputs=12
  Bus Creator1 : BusCreator  Inputs=12
  Bus Creator2 : BusCreator  Inputs=6
  Bus Creator3 : BusCreator  Inputs=6
  Bus Creator4 : BusCreator  Inputs=4
  Demux : Demux  Outputs=12
  Demux1 : Demux  Outputs=6
  Demux2 : Demux  Outputs=6
  Demux3 : Demux
  Demux4 : Demux  Outputs=12
  Kinetics : S-Function  FunctionName=TM_Sfun  Parameters='Kinetics'  SFunctionDeploymentMode=off  EnableBusSupport=off
  TireFL.Out : Ground
  TireFR.Out : Ground
  TireRL.Out : Ground
  TireRR.Out : Ground
  Sync_Out : Outport
  Trailer.Load : Outport  Port=2
  Car.Hitch : Outport  Port=3
  Car.Fr1 : Outport  Port=4
  Car.Trq_T2W : Outport  Port=5
  WheelCarrier.Misc : Outport  Port=6
  wires:
  Demux4/12 -> Bus Creator/12  "Car Trq_T2WFR2"
  Demux4/11 -> Bus Creator/11  "Car Trq_T2WFL2"
  Sync_In/1 -> Kinetics/1
  Kinetics/1 -> Sync_Out/1
  Car.Aero/1 -> Kinetics/3
  Car.Virtual/1 -> Kinetics/2
  Bus Creator1/1 -> Trailer.Load/1
  Demux/1 -> Bus Creator1/1  "Trailer Load_0 mass"
  Demux/2 -> Bus Creator1/2  "Trailer Load_0 tx"
  Demux/3 -> Bus Creator1/3  "Trailer Load_0 ty"
  Demux/4 -> Bus Creator1/4  "Trailer Load_0 tz"
  Kinetics/2 -> Demux/1
  Demux/5 -> Bus Creator1/5  "Trailer Load_1 mass"
  Demux/6 -> Bus Creator1/6  "Trailer Load_1 tx"
  Demux/7 -> Bus Creator1/7  "Trailer Load_1 ty"
  Demux/8 -> Bus Creator1/8  "Trailer Load_1 tz"
  Demux/9 -> Bus Creator1/9  "Trailer Load_2 mass"
  Demux/10 -> Bus Creator1/10  "Trailer Load_2 tx"
  Demux/11 -> Bus Creator1/11  "Trailer Load_2 ty"
  Demux/12 -> Bus Creator1/12  "Trailer Load_2 tz"
  Demux1/1 -> Bus Creator2/1  "Car Hitch tx"
  Demux1/2 -> Bus Creator2/2  "Car Hitch ty"
  Demux1/3 -> Bus Creator2/3  "Car Hitch tz"
  Demux1/4 -> Bus Creator2/4  "Car Hitch vx"
  Demux1/5 -> Bus Creator2/5  "Car Hitch vy"
  Demux1/6 -> Bus Creator2/6  "Car Hitch vz"
  Kinetics/3 -> Demux1/1
  Bus Creator2/1 -> Car.Hitch/1
  Demux2/1 -> Bus Creator3/1  "Car Fr1 rx"
  Demux2/2 -> Bus Creator3/2  "Car Fr1 ry"
  Demux2/3 -> Bus Creator3/3  "Car Fr1 rz"
  Demux2/4 -> Bus Creator3/4  "Car Fr1 rvx"
  Demux2/5 -> Bus Creator3/5  "Car Fr1 rvy"
  Demux2/6 -> Bus Creator3/6  "Car Fr1 rvz"
  Bus Creator3/1 -> Car.Fr1/1
  Kinetics/4 -> Demux2/1
  Car.Load/1 -> Kinetics/4
  Demux3/1 -> Bus Creator4/1  "car Susp FL GenInert2"
  Demux3/2 -> Bus Creator4/2  "car Susp FR GenInert2"
  Demux3/3 -> Bus Creator4/3  "car Susp FL GenFrc2"
  Demux3/4 -> Bus Creator4/4  "car Susp FR GenFrc2"
  Bus Creator4/1 -> WheelCarrier.Misc/1
  Demux4/3 -> Bus Creator/3  "Car Trq_T2WRL"
  Demux4/2 -> Bus Creator/2  "Car Trq_T2WFR"
  Demux4/1 -> Bus Creator/1  "Car Trq_T2WFL"
  TireFL.Out/1 -> Kinetics/5
  TireFR.Out/1 -> Kinetics/6
  TireRL.Out/1 -> Kinetics/7
  TireRR.Out/1 -> Kinetics/8
  FSpring_ext/1 -> Kinetics/9
  FDamp_ext/1 -> Kinetics/10
  FStabi_ext/1 -> Kinetics/11
  Kinetics/6 -> Demux3/1
  Kinetics/5 -> Demux4/1
  Bus Creator/1 -> Car.Trq_T2W/1
  Demux4/9 -> Bus Creator/9  "Car Trq_T2WRR2"
  Demux4/10 -> Bus Creator/10  "Car Trq_T2WRR2Twin"
  Demux4/7 -> Bus Creator/7  "Car Trq_T2WRL2"
  Demux4/8 -> Bus Creator/8  "Car Trq_T2WRL2Twin"
  Demux4/5 -> Bus Creator/5  "Car Trq_T2WRR"
  Demux4/4 -> Bus Creator/4  "Car Trq_T2WRLTwin"
  Demux4/6 -> Bus Creator/6  "Car Trq_T2WRRTwin"
  FBuf_ext/1 -> Kinetics/12

== system generic_truck/TruckMaker/IPG Vehicle/CarAndTrailer/Steering ==
  note: When replacing the entire steering system,
      | be sure to disable the IPG steering model by using the steering
      | model 'Model Manager off' in the vehicle GUI.
  Sync_In : Inport
  VhclCtrl.Steering : Inport  Port=2
  Bus Creator1 : BusCreator  Inputs=16
  Bus Creator2 : BusCreator  Inputs=5
  Demux : Demux  Outputs=21
  Steering : S-Function  FunctionName=TM_Sfun  Parameters='Steering'  SFunctionDeploymentMode=off  EnableBusSupport=off
  Terminator : Terminator
  Sync_Out : Outport
  Steer.IF : Outport  Port=2
  wires:
  Demux/21 -> Bus Creator2/5  "Steering IF R Inert"
  Demux/20 -> Bus Creator2/4  "Steering IF R Frc"
  Demux/19 -> Bus Creator2/3  "Steering IF L Inert"
  Demux/18 -> Bus Creator2/2  "Steering IF L Frc"
  Demux/17 -> Bus Creator2/1  "Steering IF SteerByTrq"
  Demux/16 -> Bus Creator1/16  "Steering IF R iSteer2q"
  Demux/15 -> Bus Creator1/15  "Steering IF R qpp"
  Demux/14 -> Bus Creator1/14  "Steering IF R qp"
  Demux/13 -> Bus Creator1/13  "Steering IF R q"
  Demux/12 -> Bus Creator1/12  "Steering IF L iSteer2q"
  Demux/11 -> Bus Creator1/11  "Steering IF L qpp"
  Demux/10 -> Bus Creator1/10  "Steering IF L qp"
  Demux/9 -> Bus Creator1/9  "Steering IF L q"
  Demux/8 -> Bus Creator1/8  "Steering IF AssistTrqPin"
  Demux/7 -> Bus Creator1/7  "Steering IF AssistTrqCol"
  Demux/6 -> Bus Creator1/6  "Steering IF AssistFrc"
  Demux/5 -> Bus Creator1/5  "Steering IF TrqStatic"
  Demux/4 -> Bus Creator1/4  "Steering IF Trq"
  Demux/3 -> Bus Creator1/3  "Steering IF AngAcc"
  Demux/2 -> Bus Creator1/2  "Steering IF AngVel"
  Demux/1 -> Bus Creator1/1  "Steering IF Ang"
  Bus Creator1/1 -> Steer.IF/1
  Bus Creator2/1 -> Terminator/1  "Steer IF (in)"
  Sync_In/1 -> Steering/1
  Steering/1 -> Sync_Out/1
  VhclCtrl.Steering/1 -> Steering/2
  Steering/2 -> Demux/1

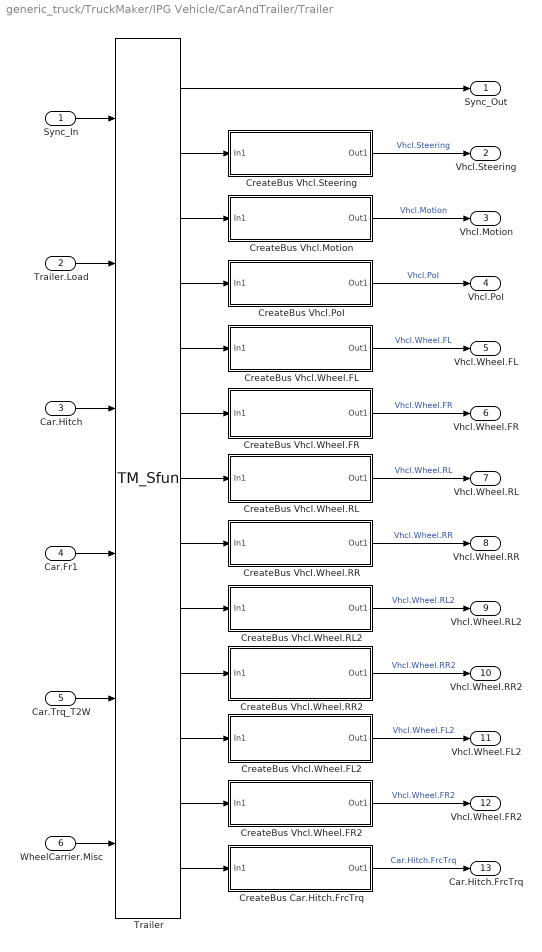
== system generic_truck/TruckMaker/IPG Vehicle/CarAndTrailer/Trailer ==
  Sync_In : Inport
  Trailer.Load : Inport  Port=2
  Car.Hitch : Inport  Port=3
  Car.Fr1 : Inport  Port=4
  Car.Trq_T2W : Inport  Port=5
  WheelCarrier.Misc : Inport  Port=6
  CreateBus Car.Hitch.FrcTrq : Subsystem
  CreateBus Vhcl.Motion : Subsystem
  CreateBus Vhcl.PoI : Subsystem
  CreateBus Vhcl.Steering : Subsystem
  CreateBus Vhcl.Wheel.FL : Subsystem
  CreateBus Vhcl.Wheel.FL2 : Subsystem
  CreateBus Vhcl.Wheel.FR : Subsystem
  CreateBus Vhcl.Wheel.FR2 : Subsystem
  CreateBus Vhcl.Wheel.RL : Subsystem
  CreateBus Vhcl.Wheel.RL2 : Subsystem
  CreateBus Vhcl.Wheel.RR : Subsystem
  CreateBus Vhcl.Wheel.RR2 : Subsystem
  Trailer : S-Function  FunctionName=TM_Sfun  Parameters='Trailer'  SFunctionDeploymentMode=off  EnableBusSupport=off
  Sync_Out : Outport
  Vhcl.Steering : Outport  Port=2
  Vhcl.Motion : Outport  Port=3
  Vhcl.PoI : Outport  Port=4
  Vhcl.Wheel.FL : Outport  Port=5
  Vhcl.Wheel.FR : Outport  Port=6
  Vhcl.Wheel.RL : Outport  Port=7
  Vhcl.Wheel.RR : Outport  Port=8
  Vhcl.Wheel.RL2 : Outport  Port=9
  Vhcl.Wheel.RR2 : Outport  Port=10
  Vhcl.Wheel.FL2 : Outport  Port=11
  Vhcl.Wheel.FR2 : Outport  Port=12
  Car.Hitch.FrcTrq : Outport  Port=13
  wires:
  CreateBus Vhcl.Wheel.RL2/1(Out1) -> Vhcl.Wheel.RL2/1  "Vhcl.Wheel.RL2"
  CreateBus Vhcl.Wheel.RR2/1(Out1) -> Vhcl.Wheel.RR2/1  "Vhcl.Wheel.RR2"
  CreateBus Vhcl.Wheel.FL2/1(Out1) -> Vhcl.Wheel.FL2/1  "Vhcl.Wheel.FL2"
  CreateBus Vhcl.Wheel.FR2/1(Out1) -> Vhcl.Wheel.FR2/1  "Vhcl.Wheel.FR2"
  Trailer/12 -> CreateBus Vhcl.Wheel.FR2/1(In1)
  Trailer/11 -> CreateBus Vhcl.Wheel.FL2/1(In1)
  Trailer/10 -> CreateBus Vhcl.Wheel.RR2/1(In1)
  Trailer/9 -> CreateBus Vhcl.Wheel.RL2/1(In1)
  CreateBus Vhcl.Wheel.FL/1(Out1) -> Vhcl.Wheel.FL/1  "Vhcl.Wheel.FL"
  CreateBus Vhcl.Wheel.FR/1(Out1) -> Vhcl.Wheel.FR/1  "Vhcl.Wheel.FR"
  CreateBus Vhcl.Wheel.RL/1(Out1) -> Vhcl.Wheel.RL/1  "Vhcl.Wheel.RL"
  CreateBus Vhcl.Wheel.RR/1(Out1) -> Vhcl.Wheel.RR/1  "Vhcl.Wheel.RR"
  Trailer/8 -> CreateBus Vhcl.Wheel.RR/1(In1)
  Trailer/7 -> CreateBus Vhcl.Wheel.RL/1(In1)
  Trailer/6 -> CreateBus Vhcl.Wheel.FR/1(In1)
  Trailer/5 -> CreateBus Vhcl.Wheel.FL/1(In1)
  Trailer/13 -> CreateBus Car.Hitch.FrcTrq/1(In1)
  Trailer/2 -> CreateBus Vhcl.Steering/1(In1)
  CreateBus Vhcl.Steering/1(Out1) -> Vhcl.Steering/1  "Vhcl.Steering"
  Trailer/3 -> CreateBus Vhcl.Motion/1(In1)
  Trailer/4 -> CreateBus Vhcl.PoI/1(In1)
  CreateBus Vhcl.PoI/1(Out1) -> Vhcl.PoI/1  "Vhcl.PoI"
  CreateBus Vhcl.Motion/1(Out1) -> Vhcl.Motion/1  "Vhcl.Motion"
  Car.Trq_T2W/1 -> Trailer/5
  WheelCarrier.Misc/1 -> Trailer/6
  CreateBus Car.Hitch.FrcTrq/1(Out1) -> Car.Hitch.FrcTrq/1  "Car.Hitch.FrcTrq"
  Car.Fr1/1 -> Trailer/4
  Car.Hitch/1 -> Trailer/3
  Trailer.Load/1 -> Trailer/2
  Trailer/1 -> Sync_Out/1
  Sync_In/1 -> Trailer/1

== system generic_truck/TruckMaker/IPG Vehicle/CarAndTrailer/CarAndTrailerUpd/CreateBus Brake.IF.In ==
  In : Inport
  BusCreator : BusCreator  Inputs=17
  Demux : Demux  Outputs=17
  Out : Outport
  wires:
  Demux/17 -> BusCreator/17  "Brake IF Trq_Reg FR2"
  Demux/16 -> BusCreator/16  "Brake IF Trq_Reg FL2"
  Demux/15 -> BusCreator/15  "Brake IF Trq_Reg RR2"
  Demux/14 -> BusCreator/14  "Brake IF Trq_Reg RL2"
  Demux/13 -> BusCreator/13  "Brake IF Trq_Reg RR"
  Demux/12 -> BusCreator/12  "Brake IF Trq_Reg RL"
  Demux/11 -> BusCreator/11  "Brake IF Trq_Reg FR"
  Demux/10 -> BusCreator/10  "Brake IF Trq_Reg FL"
  Demux/9 -> BusCreator/9  "Brake IF Trq_Reg_max FR2"
  Demux/8 -> BusCreator/8  "Brake IF Trq_Reg_max FL2"
  Demux/7 -> BusCreator/7  "Brake IF Trq_Reg_max RR2"
  Demux/6 -> BusCreator/6  "Brake IF Trq_Reg_max RL2"
  Demux/5 -> BusCreator/5  "Brake IF Trq_Reg_max RR"
  Demux/4 -> BusCreator/4  "Brake IF Trq_Reg_max RL"
  Demux/3 -> BusCreator/3  "Brake IF Trq_Reg_max FR"
  Demux/2 -> BusCreator/2  "Brake IF Trq_Reg_max FL"
  Demux/1 -> BusCreator/1  "Brake IF T_env"
  BusCreator/1 -> Out/1
  In/1 -> Demux/1

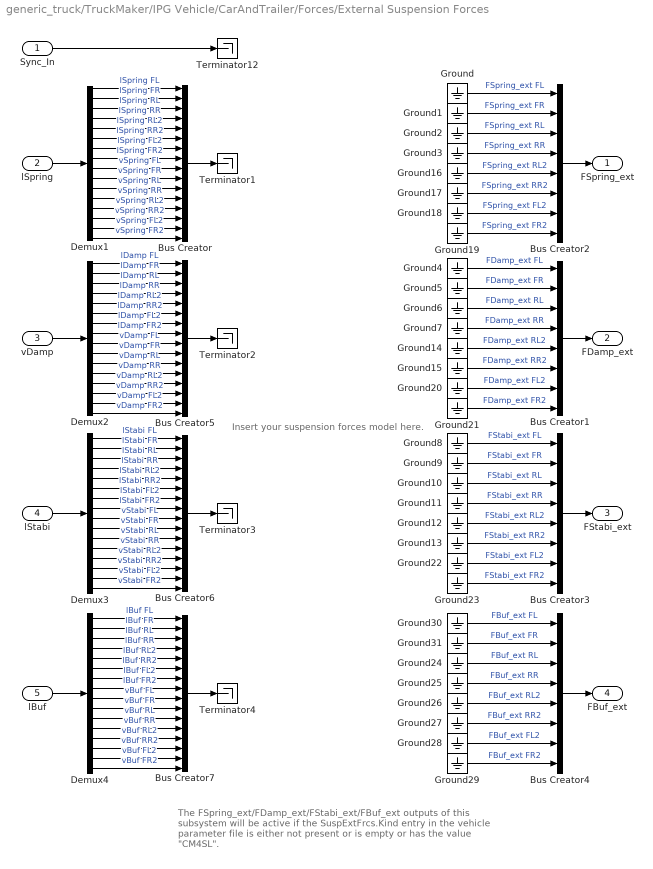
== system generic_truck/TruckMaker/IPG Vehicle/CarAndTrailer/Forces/External Suspension Forces ==
  note: The FSpring_ext/FDamp_ext/FStabi_ext/FBuf_ext outputs of this subsystem will be
      | active if the SuspExtFrcs.Kind entry in the vehicle parameter file
      | is either not present or is empty or has the value "CM4SL".
  note: Insert your suspension forces model here.
  Sync_In : Inport
  lSpring : Inport  Port=2
  vDamp : Inport  Port=3
  lStabi : Inport  Port=4
  lBuf : Inport  Port=5
  Bus Creator{,5..7} (4 alike) : BusCreator  Inputs=16
  Bus Creator{1..4} (4 alike) : BusCreator  Inputs=8
  Demux{1..4} (4 alike) : Demux  Outputs=16
  Ground{,1..31} (32 alike) : Ground
  Terminator{1..4,12} (5 alike) : Terminator
  FSpring_ext : Outport
  FDamp_ext : Outport  Port=2
  FStabi_ext : Outport  Port=3
  FBuf_ext : Outport  Port=4
  wires:
  Demux3/10 -> Bus Creator6/10  "vStabi FR"
  Demux4/16 -> Bus Creator7/16  "vBuf FR2"
  Demux4/15 -> Bus Creator7/15  "vBuf FL2"
  Demux4/14 -> Bus Creator7/14  "vBuf RR2"
  Demux4/13 -> Bus Creator7/13  "vBuf RL2"
  Demux4/12 -> Bus Creator7/12  "vBuf RR"
  Demux4/11 -> Bus Creator7/11  "vBuf RL"
  Demux4/10 -> Bus Creator7/10  "vBuf FR"
  Demux4/9 -> Bus Creator7/9  "vBuf FL"
  Demux3/16 -> Bus Creator6/16  "vStabi FR2"
  Demux3/15 -> Bus Creator6/15  "vStabi FL2"
  Demux3/14 -> Bus Creator6/14  "vStabi RR2"
  Demux3/13 -> Bus Creator6/13  "vStabi RL2"
  Demux3/12 -> Bus Creator6/12  "vStabi RR"
  Demux3/11 -> Bus Creator6/11  "vStabi RL"
  Demux3/9 -> Bus Creator6/9  "vStabi FL"
  Bus Creator6/1 -> Terminator3/1
  Bus Creator7/1 -> Terminator4/1
  Bus Creator5/1 -> Terminator2/1
  Bus Creator/1 -> Terminator1/1
  Demux2/16 -> Bus Creator5/16  "vDamp FR2"
  Demux2/15 -> Bus Creator5/15  "vDamp FL2"
  Demux2/14 -> Bus Creator5/14  "vDamp RR2"
  Demux2/13 -> Bus Creator5/13  "vDamp RL2"
  Demux2/12 -> Bus Creator5/12  "vDamp RR"
  Demux2/11 -> Bus Creator5/11  "vDamp RL"
  Demux2/10 -> Bus Creator5/10  "vDamp FR"
  Demux2/9 -> Bus Creator5/9  "vDamp FL"
  Demux1/16 -> Bus Creator/16  "vSpring FR2"
  Demux1/15 -> Bus Creator/15  "vSpring FL2"
  Demux1/14 -> Bus Creator/14  "vSpring RR2"
  Demux1/13 -> Bus Creator/13  "vSpring RL2"
  Demux1/12 -> Bus Creator/12  "vSpring RR"
  Demux1/11 -> Bus Creator/11  "vSpring RL"
  Demux1/10 -> Bus Creator/10  "vSpring FR"
  Demux1/9 -> Bus Creator/9  "vSpring FL"
  Demux3/7 -> Bus Creator6/7  "lStabi FL2"
  Demux3/8 -> Bus Creator6/8  "lStabi FR2"
  Ground22/1 -> Bus Creator3/7  "FStabi_ext FL2"
  Ground23/1 -> Bus Creator3/8  "FStabi_ext FR2"
  Demux2/7 -> Bus Creator5/7  "lDamp FL2"
  Demux2/8 -> Bus Creator5/8  "lDamp FR2"
  Ground20/1 -> Bus Creator1/7  "FDamp_ext FL2"
  Ground21/1 -> Bus Creator1/8  "FDamp_ext FR2"
  Ground18/1 -> Bus Creator2/7  "FSpring_ext FL2"
  Ground19/1 -> Bus Creator2/8  "FSpring_ext FR2"
  Demux1/7 -> Bus Creator/7  "lSpring FL2"
  Demux1/8 -> Bus Creator/8  "lSpring FR2"
  Sync_In/1 -> Terminator12/1
  lSpring/1 -> Demux1/1
  vDamp/1 -> Demux2/1
  lStabi/1 -> Demux3/1
  Demux3/1 -> Bus Creator6/1  "lStabi FL"
  Demux3/2 -> Bus Creator6/2  "lStabi FR"
  Demux3/3 -> Bus Creator6/3  "lStabi RL"
  Demux3/4 -> Bus Creator6/4  "lStabi RR"
  Demux1/1 -> Bus Creator/1  "lSpring FL"
  Demux1/2 -> Bus Creator/2  "lSpring FR"
  Demux1/3 -> Bus Creator/3  "lSpring RL"
  Demux1/4 -> Bus Creator/4  "lSpring RR"
  Demux2/1 -> Bus Creator5/1  "lDamp FL"
  Demux2/2 -> Bus Creator5/2  "lDamp FR"
  Demux2/3 -> Bus Creator5/3  "lDamp RL"
  Demux2/4 -> Bus Creator5/4  "lDamp RR"
  Bus Creator2/1 -> FSpring_ext/1
  Ground/1 -> Bus Creator2/1  "FSpring_ext FL"
  Ground1/1 -> Bus Creator2/2  "FSpring_ext FR"
  Ground2/1 -> Bus Creator2/3  "FSpring_ext RL"
  Ground3/1 -> Bus Creator2/4  "FSpring_ext RR"
  Ground4/1 -> Bus Creator1/1  "FDamp_ext FL"
  Ground5/1 -> Bus Creator1/2  "FDamp_ext FR"
  Ground6/1 -> Bus Creator1/3  "FDamp_ext RL"
  Ground7/1 -> Bus Creator1/4  "FDamp_ext RR"
  Bus Creator1/1 -> FDamp_ext/1
  Ground8/1 -> Bus Creator3/1  "FStabi_ext FL"
  Ground9/1 -> Bus Creator3/2  "FStabi_ext FR"
  Ground10/1 -> Bus Creator3/3  "FStabi_ext RL"
  Ground11/1 -> Bus Creator3/4  "FStabi_ext RR"
  Bus Creator3/1 -> FStabi_ext/1
  Demux3/5 -> Bus Creator6/5  "lStabi RL2"
  Demux3/6 -> Bus Creator6/6  "lStabi RR2"
  Ground12/1 -> Bus Creator3/5  "FStabi_ext RL2"
  Ground13/1 -> Bus Creator3/6  "FStabi_ext RR2"
  Demux2/5 -> Bus Creator5/5  "lDamp RL2"
  Demux2/6 -> Bus Creator5/6  "lDamp RR2"
  Ground14/1 -> Bus Creator1/5  "FDamp_ext RL2"
  Ground15/1 -> Bus Creator1/6  "FDamp_ext RR2"
  Demux1/5 -> Bus Creator/5  "lSpring RL2"
  Demux1/6 -> Bus Creator/6  "lSpring RR2"
  Ground16/1 -> Bus Creator2/5  "FSpring_ext RL2"
  Ground17/1 -> Bus Creator2/6  "FSpring_ext RR2"
  Demux4/7 -> Bus Creator7/7  "lBuf FL2"
  Demux4/8 -> Bus Creator7/8  "lBuf FR2"
  Ground28/1 -> Bus Creator4/7  "FBuf_ext FL2"
  Ground29/1 -> Bus Creator4/8  "FBuf_ext FR2"
  lBuf/1 -> Demux4/1
  Demux4/1 -> Bus Creator7/1  "lBuf FL"
  Demux4/2 -> Bus Creator7/2  "lBuf FR"
  Demux4/3 -> Bus Creator7/3  "lBuf RL"
  Demux4/4 -> Bus Creator7/4  "lBuf RR"
  Ground30/1 -> Bus Creator4/1  "FBuf_ext FL"
  Ground31/1 -> Bus Creator4/2  "FBuf_ext FR"
  Ground24/1 -> Bus Creator4/3  "FBuf_ext RL"
  Ground25/1 -> Bus Creator4/4  "FBuf_ext RR"
  Bus Creator4/1 -> FBuf_ext/1
  Demux4/5 -> Bus Creator7/5  "lBuf RL2"
  Demux4/6 -> Bus Creator7/6  "lBuf RR2"
  Ground26/1 -> Bus Creator4/5  "FBuf_ext RL2"
  Ground27/1 -> Bus Creator4/6  "FBuf_ext RR2"
